simulink model "TAYLOR_TYPE_ZNNK"  (R2024a)
settings: Solver=ode4  StartTime=0.0  StopTime=10.0  FixedStep=0.01  RelTol=1e-3
values from neighbouring files (symbols this model uses):
  h = tau*gamma    (= 0.4)    [setup.m]
  tau = 0.01    [setup.m]
  y0 = ones(3, 1)    [setup.m]
  y1 = ones(3, 1)    [setup.m]
  y2 = ones(3, 1)    [setup.m]
settings Model: Creator=uli_2  LastModifiedBy=uli_2
settings DebuggingCC: UnconnectedInputMsg=warning  UnconnectedOutputMsg=warning  UnconnectedLineMsg=warning
settings ModelReferenceCC: EnableRefExpFcnMdlSchedulingChecks=on
settings RTWCC: GPUComputeCapability=3.5  DLArmComputeVersion=19.05

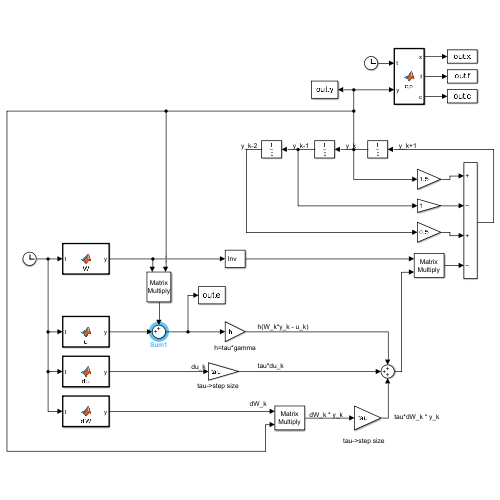
[thumbnail: Simulink's stored preview of the top-level diagram]
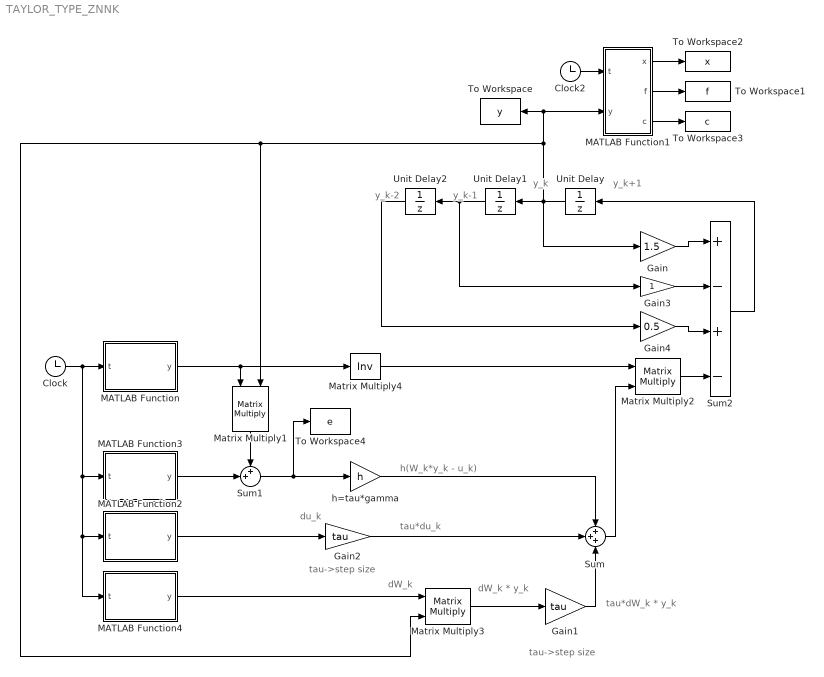
== system TAYLOR_TYPE_ZNNK ==
  note: tau*du_k
  note: dW_k
  note: tau->step size
  note: tau*dW_k * y_k
  note: y_k+1
  note: du_k
  note: y_k
  note: h(W_k*y_k - u_k)
  note: dW_k * y_k
  note: tau->step size
  note: y_k-1
  note: y_k-2
  Clock : Clock
  Clock2 : Clock
  Gain : Gain  Gain=1.5
  Gain1 : Gain  Gain=tau
  Gain2 : Gain  Gain=tau
  Gain3 : Gain
  Gain4 : Gain  Gain=0.5
  MATLAB Function : MATLAB Function  TreatAsAtomicUnit=on
  MATLAB Function1 : MATLAB Function  TreatAsAtomicUnit=on
  MATLAB Function2 : MATLAB Function  TreatAsAtomicUnit=on
  MATLAB Function3 : MATLAB Function  TreatAsAtomicUnit=on
  MATLAB Function4 : MATLAB Function  TreatAsAtomicUnit=on
  Matrix Multiply1 : Product  Multiplication=Matrix(*)
  Matrix Multiply2 : Product  Multiplication=Matrix(*)
  Matrix Multiply3 : Product  Multiplication=Matrix(*)
  Matrix Multiply4 : Product  Inputs=/  Multiplication=Matrix(*)
  Sum : Sum  Inputs=+++
  Sum1 : Sum  Inputs=++|
  Sum2 : Sum  Inputs=+-+-
  To Workspace : ToWorkspace  VariableName=y  SaveFormat=Timeseries  SampleTime=-1
  To Workspace1 : ToWorkspace  VariableName=f  SaveFormat=Timeseries  SampleTime=-1
  To Workspace2 : ToWorkspace  VariableName=x  SaveFormat=Timeseries  SampleTime=-1
  To Workspace3 : ToWorkspace  VariableName=c  SaveFormat=Timeseries  SampleTime=-1
  To Workspace4 : ToWorkspace  VariableName=e  SaveFormat=Timeseries  SampleTime=-1
  Unit Delay : UnitDelay  InitialCondition=y2  SampleTime=-1  HasFrameUpgradeWarning=on
  Unit Delay1 : UnitDelay  InitialCondition=y1  SampleTime=-1  HasFrameUpgradeWarning=on
  Unit Delay2 : UnitDelay  InitialCondition=y0  SampleTime=-1  HasFrameUpgradeWarning=on
  h=tau*gamma : Gain  Gain=h
  wires:
  Unit Delay/1 -> Gain/1, MATLAB Function1/2(y), To Workspace/1, Matrix Multiply1/2, Matrix Multiply3/2, Unit Delay1/1
  MATLAB Function1/2(f) -> To Workspace1/1
  MATLAB Function1/1(x) -> To Workspace2/1
  MATLAB Function2/1(y) -> Gain2/1
  Matrix Multiply3/1 -> Gain1/1
  Sum1/1 -> To Workspace4/1, h=tau*gamma/1
  MATLAB Function1/3(c) -> To Workspace3/1
  MATLAB Function/1(y) -> Matrix Multiply4/1, Matrix Multiply1/1
  Matrix Multiply1/1 -> Sum1/1
  MATLAB Function3/1(y) -> Sum1/2
  MATLAB Function4/1(y) -> Matrix Multiply3/1
  Clock/1 -> MATLAB Function4/1(t), MATLAB Function2/1(t), MATLAB Function3/1(t), MATLAB Function/1(t)
  Unit Delay1/1 -> Gain3/1, Unit Delay2/1
  Gain1/1 -> Sum/3
  Gain2/1 -> Sum/2
  h=tau*gamma/1 -> Sum/1
  Matrix Multiply4/1 -> Matrix Multiply2/1
  Sum/1 -> Matrix Multiply2/2
  Clock2/1 -> MATLAB Function1/1(t)
  Matrix Multiply2/1 -> Sum2/4
  Gain/1 -> Sum2/1
  Gain3/1 -> Sum2/2
  Gain4/1 -> Sum2/3
  Unit Delay2/1 -> Gain4/1
  Sum2/1 -> Unit Delay/1

== matlab function TAYLOR_TYPE_ZNNK/MATLAB Function1 ==
  data: t input; y input; x output; f output; c output
function [x,f,c] = qp(t, y)
    n = 2;
    x = y(1:n); lambda = y(n+1:end);
    P = [sin(t)/4 + 1, cos(t)/2; cos(t)/2, cos(t)/4 + 1];
    A = [sin(4*t), cos(4*t)];
    q = [sin(3*t); cos(3*t)];
    b = cos(2*t);
    f = x' * P * x + q' * x;
    c = A * x - b;

== matlab function TAYLOR_TYPE_ZNNK/MATLAB Function ==
  data: t input; y output
function y = W(t)
    m = 1;
    P = [sin(t)/4 + 1, cos(t)/2; cos(t)/2, cos(t)/4 + 1];
    A = [sin(4*t), cos(4*t)];
    y = [P, A'; A, zeros(m)];

== matlab function TAYLOR_TYPE_ZNNK/MATLAB Function2 ==
  data: t input; y output
function y = du(t)
    y = [3*cos(3*t); -3*sin(3*t); 2*sin(2*t)];

== matlab function TAYLOR_TYPE_ZNNK/MATLAB Function3 ==
  data: t input; y output
function y = u(t)
    q = [sin(3*t); cos(3*t)];
    b = cos(2*t);
    y = [q; -b];

== matlab function TAYLOR_TYPE_ZNNK/MATLAB Function4 ==
  data: t input; y output
function y = dW(t)
    m = 1;
    dP = [cos(t)/4, -sin(t)/2; -sin(t)/2, -sin(t)/4];
    dA = [4*cos(4*t), -4*sin(4*t)];
    y = [dP, dA'; dA, zeros(m)];
